simulink model "srrc_filter_model"  (R2020b)
settings: Solver=FixedStepDiscrete  StartTime=0.0  StopTime=20  RelTol=1e-3
undefined symbols (not defined in the file or in its folder): srrc_trans_coeffs
libraries: hdlsllib x3, simulink x1
settings Model: DataTypeOverride=Off  Creator=wardo  LastModifiedBy=wardo
settings DataIOCC: LimitDataPoints=on  SaveOutput=off  SaveTime=off
settings OptimizationCC: BlockReduction=off  ConditionallyExecuteInputs=off  DefaultParameterBehavior=Inlined  LifeSpan=inf
settings DebuggingCC: AlgebraicLoopMsg=error  SingleTaskRateTransMsg=error  AllowSymbolicDim=off  StrictBusMsg=ErrorOnBusTreatedAsVector  SFUnexpectedBacktrackingDiag=warning  SFNoUnconditionalDefaultTransitionDiag=warning  SFExecutionAtInitializationDiag=none  ArithmeticOperatorsInVariantConditions=warning
settings HardwareCC: ProdBitPerPointer=32  ProdBitPerSizeT=32  ProdBitPerPtrDiffT=32  ProdLargestAtomicFloat=None  ProdIntDivRoundTo=Undefined  ProdEndianess=Unspecified  ProdWordSize=32  ProdHWDeviceType=ASIC/FPGA->ASIC/FPGA  ProdEqTarget=off
settings SFSimCC: SimUseLocalCustomCode=off  CustomCodeUndefinedFunction=UseInterfaceOnly
settings RTWCC: RTWUseLocalCustomCode=off
settings CodeAppCC: StateflowObjectComments=on
settings GRTTargetCC: TargetLangStandard=C89/C90 (ANSI)
settings ConfigComp: CovScope=ReferencedModels  CovMetricSettings=dw  CovSaveCumulativeToWorkspaceVar=on  CovSaveSingleToWorkspaceVar=on  CovExternalEMLEnable=off  CovSFcnEnable=off

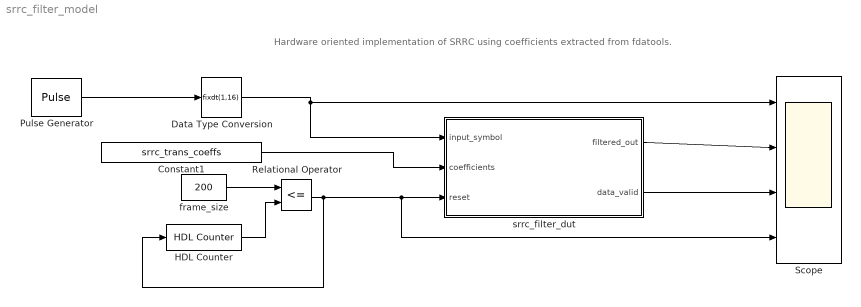
== system srrc_filter_model ==
  note: Hardware oriented implementation of SRRC using coefficients extracted from fdatools.
  Constant1 : Constant  Value=srrc_trans_coeffs  SampleTime=-1
  Data Type Conversion : DataTypeConversion  OutMin=0  OutMax=5  OutDataTypeStr=fixdt(1,16)  RndMeth=Nearest
  HDL Counter : hdlsllib/Sources/HDL Counter  CountType=Free running  CountInit=0  CountStep=1  CountMax=100  CountFromType=Initial value  CountFrom=0  CountResetPort=on  CountLoadPort=off  CountEnbPort=off  CountDirPort=off  CountDataType=Unsigned  CountWordLen=8  CountFracLen=0  CountSampTime=1
  Pulse Generator : DiscretePulseGenerator  PulseType=Time based  Amplitude=5  Period=2.5
  Relational Operator : RelationalOperator  Operator=<=  OutDataTypeStr=boolean  RndMeth=Nearest
  Scope : Scope  NumInputPorts=4
  frame_size : Constant  Value=200  SampleTime=-1
  srrc_filter_dut : Subsystem
  wires:
  Pulse Generator/1 -> Data Type Conversion/1
  srrc_filter_dut/1(filtered_out) -> Scope/2
  Constant1/1 -> srrc_filter_dut/2(coefficients)
  Data Type Conversion/1 -> srrc_filter_dut/1(input_symbol), Scope/1
  srrc_filter_dut/2(data_valid) -> Scope/3
  HDL Counter/1 -> Relational Operator/2
  frame_size/1 -> Relational Operator/1
  Relational Operator/1 -> HDL Counter/1, Scope/4, srrc_filter_dut/3(reset)

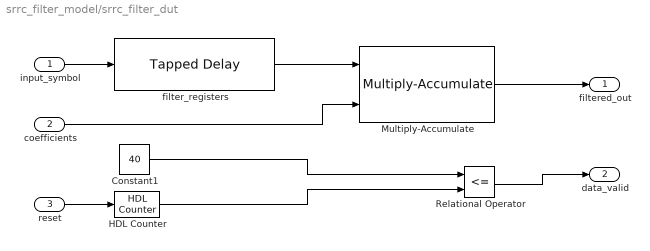
== system srrc_filter_model/srrc_filter_dut ==
  input_symbol : Inport
  coefficients : Inport  Port=2
  reset : Inport  Port=3
  Constant1 : Constant  Value=40  SampleTime=-1
  HDL Counter : hdlsllib/Sources/HDL Counter  CountType=Free running  CountInit=0  CountStep=1  CountMax=40  CountFromType=Initial value  CountFrom=0  CountResetPort=on  CountLoadPort=off  CountEnbPort=off  CountDirPort=off  CountDataType=Unsigned  CountWordLen=8  CountFracLen=0  CountSampTime=1
  Multiply-Accumulate : hdlsllib/HDL Operations/Multiply-Accumulate  opMode=Vector  initValueSetting=Dialog  initValue=0  initValueSetting2=Dialog  initValue2=0  initValueSetting3=Dialog  initValue3=0  num_samples=2  RndMeth=Nearest  RndMeth2=Floor  RndMeth3=Floor  datatype2=Inherit: Inherit via back propagation  datatype3=Inherit: Inherit via back propagation  validOut=on  endInandOut=on  startOut=on  countOut=on  dim=-1  DoSatur=off  parallel=off
      settings: SourceProductBaseCode=SL
  Relational Operator : RelationalOperator  Operator=<=  OutDataTypeStr=boolean  RndMeth=Nearest
  filter_registers : simulink/Discrete/Tapped Delay  vinit=0.0  samptime=-1  NumDelays=80  DelayOrder=Oldest  includeCurrent=on
  filtered_out : Outport  VectorParamsAs1DForOutWhenUnconnected=off
  data_valid : Outport  Port=2  VectorParamsAs1DForOutWhenUnconnected=off
  wires:
  Multiply-Accumulate/1 -> filtered_out/1
  filter_registers/1 -> Multiply-Accumulate/1
  input_symbol/1 -> filter_registers/1
  coefficients/1 -> Multiply-Accumulate/2
  Constant1/1 -> Relational Operator/1
  Relational Operator/1 -> data_valid/1
  HDL Counter/1 -> Relational Operator/2
  reset/1 -> HDL Counter/1
